simulink model "os_Rcontroller"  (R2017b)
settings: Solver=VariableStepAuto  StartTime=0.0  StopTime=10.0  RelTol=1e-3
settings Model: Creator=Kalana  LastModifiedBy=Kalana

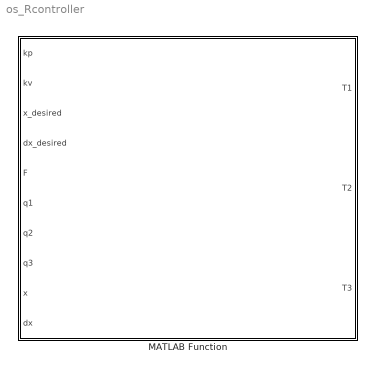
== system os_Rcontroller ==
  MATLAB Function : MATLAB Function  TreatAsAtomicUnit=on

== matlab function os_Rcontroller/MATLAB Function ==
  data: kp input; kv input; x_desired input; dx_desired input; F input; T1 output; q1 input; q2 input; q3 input; x input; dx input; T2 output; T3 output
function [T1, T2, T3] = rightLegControl(kp, kv, x_desired, dx_desired, F, q1, q2, q3, x, dx)

g = [0    ;
     0    ;
     -9.8 ];

Mass_1 = [1.13919,  0,        0;
          0,        1.13919,  0;
          0,        0,        1.13919];

Iner_1 = [ 4703123.40e-09,     -3169987.54e-09,     210.39e-09;
           -3169987.54e-09,    4976200.05e-09,     -364.11e-09;
           210.39e-09,         -364.11e-09,         8601629.18e-09];

      
Mass_2 = [1.13671,  0,        0;
          0,        1.13671,  0;
          0,        0,        1.13671];

Iner_2 = [2565673.28e-09,      32.99e-09,           2839694.73e-09;
          32.99e-09,           12592746.15e-09,     -50.96e-09;
          2839694.73e-09,      -50.96e-09,          10643810.45e-09];

      
Mass_3 = [0.63820,  0,        0;
          0,        0.63820,  0;
          0,        0,        0.63280];
  
Iner_3 = [728680.81e-09,      -172.39e-09,        158.48e-09;
          -172.39e-09,        2618699.35e-09,     -3.33e-09;
          158.48e-09,         -3.33e-09,          2391085.66e-09];

      
Jv1 = [-0.05734*cos(q1)-0.05586*sin(q1),   0, 0;
       0,                                  0, 0;
       +0.05734*sin(q1)-0.05586*cos(q1)    0, 0];

Jw1 = [0, 0, 0;
       1, 0, 0;
       0, 0, 0];

   
Jv2 = [-0.100*sin(q1)*cos(q2)-0.0773*cos(q1)-0.1225*sin(q1),  -0.100*cos(q1)*sin(q2),     0;
       0,                                                     0.100*cos(q2),              0; 
       0.100*cos(q1)*cos(q2)+0.0773*sin(q1)-0.1225*cos(q1),   -0.100*sin(q1)*sin(q2),     0]; 
      
Jw2 = [0, 1, 0; 
       1, 0, 0; 
       0, 0, 0];
 
   
Jv3 = [-0.02559*sin(q1)*cos(q2-q3)-0.2*sin(q1)*cos(q2)-0.1225*sin(q1)-0.0525*cos(q1),  -0.02559*cos(q1)*sin(q2-q3)-0.2*cos(q1)*sin(q2),  0.02559*cos(q1)*sin(q2-q3) ;
       0,                                                                              0.02559*cos(q2-q3)+0.2*cos(q2),                   -0.02559*cos(q2-q3)         ;
       -0.02559*cos(q1)*cos(q2-q3)-0.2*cos(q1)*cos(q2)-0.1225*cos(q1)+0.0525*sin(q1),  0.02559*sin(q1)*sin(q2-q3)+0.2*sin(q1)*sin(q2),   -0.02559*sin(q1)*sin(q2-q3)];
      
Jw3 = [0, 1, -1;
       1, 0,  0;
       0, 0,  0];

   
JvEE =[-0.265*sin(q1)*cos(q2-q3)-0.2*sin(q1)*cos(q2)-0.1225*sin(q1)-0.0525*cos(q1), -0.265*cos(q1)*sin(q2-q3)-0.2*cos(q1)*sin(q2),     0.265*cos(q1)*sin(q2-q3) ;
       0,                                                                           0.265*cos(q2-q3)+0.2*cos(q2),                      -0.265*cos(q2-q3)         ;
       -0.265*cos(q1)*cos(q2-q3)-0.2*cos(q1)*cos(q2)-0.1225*cos(q1)+0.0525*sin(q1), 0.265*sin(q1)*sin(q2-q3)+0.2*sin(q1)*sin(q2),      -0.265*sin(q1)*sin(q2-q3)]; 
   

Mass_q = Jv1'*Mass_1*Jv1 + Jw1'*Iner_1*Jw1 + Jv2'*Mass_2*Jv2 + Jw2'*Iner_2*Jw2 + Jv3'*Mass_3*Jv3 + Jw3'*Iner_3*Jw3;

Mass_x = JvEE'*pinv(JvEE*inv(Mass_q)*JvEE');

Grav = Jv1'*Mass_1*g + Jv2'*Mass_2*g + Jv3'*Mass_3*g;

Force = JvEE'*F;

torque = Mass_x(kp(x_desired - x) + kv(dx_desired - dx)) + Grav + Force;

T1 = torque(1);
T2 = torque(2);
T3 = torque(3);
